simulink model "Speed_control"  (R2016b)
settings: Solver=VariableStepAuto  StartTime=0.0  StopTime=3  FixedStep=5e-6  RelTol=1e-3
libraries: powerlib x6, simulink x4, powerlib_meascontrol x3
settings Model: Creator=Awab Anwar  LastModifiedBy=Awab Anwar
settings DebuggingCC: MaxConsecutiveZCsMsg=none

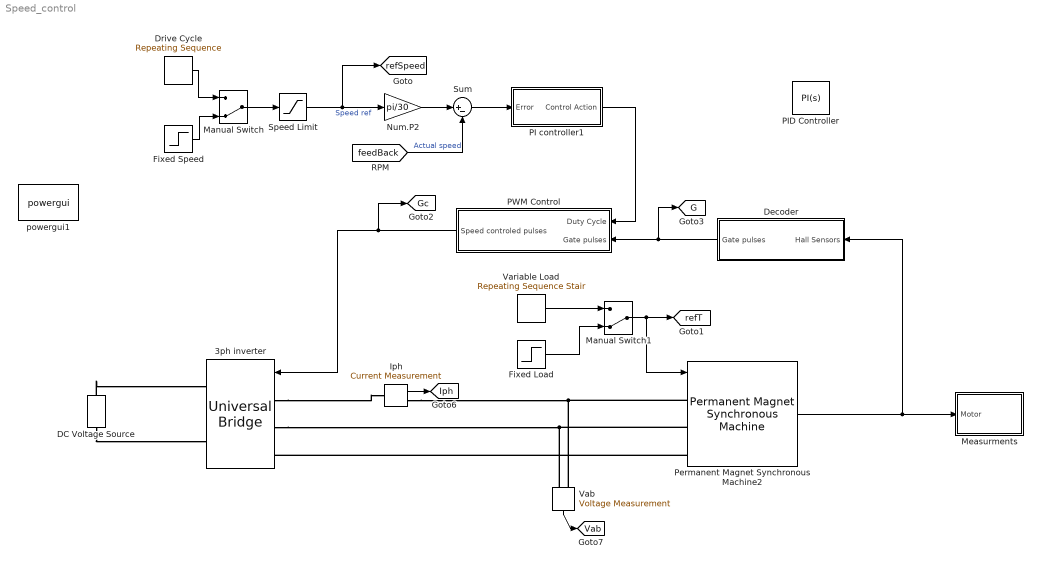
== system Speed_control ==
  3ph inverter : powerlib/Power Electronics/Universal Bridge  Arms=3  SnubberResistance=100  SnubberCapacitance=10e-6  Device=MOSFET / Diodes  Ron=0.000000001  Lon=0  ForwardVoltages="[  0  0  ]"  ForwardVoltage=0  GTOparameters=[ 10e-6 , 20e-6 ]  IGBTparameters=[ 1e-6 , 2e-6 ]  Measurements=Device voltages  Measurements_2=None  converterType=Rectifier
  DC Voltage Source : powerlib/Electrical Sources/DC Voltage Source  Amplitude=24  Measurements=None
  Decoder : Subsystem
  "Drive Cycle " : simulink/Sources/Repeating Sequence  rep_seq_t=[0 1 2 3 4 5 5.001 6 6.001 7]  rep_seq_y=[0 0 20 20 50 50 100 100 200 200]
  Fixed Speed : Step  Time=0  After=150  SampleTime=0
  Fixed Load : Step  Time=0  SampleTime=0
  Iph : powerlib/Measurements/Current Measurement  PhasorSimulation=off  OutputType=Complex  PSBequivalent=0
  Manual Switch : ManualSwitch  CurrentSetting=0
  Manual Switch1 : ManualSwitch  CurrentSetting=0
  Measurments : Subsystem
  Num.P2 : Gain  Gain=pi/30
  PI controller1 : Subsystem
  PID Controller : simulink/Continuous/PID Controller  Controller=PI  TimeDomain=Continuous-time  SampleTime=-1  IntegratorMethod=Forward Euler  FilterMethod=Forward Euler  Form=Parallel  UseFilter=on  ControllerParametersSource=internal  P=3  I=11.6  D=0  N=100  InitialConditionSource=internal  InitialConditionForIntegrator=0  InitialConditionForFilter=0  ExternalReset=none  LimitOutput=off  UpperSaturationLimit=inf  LowerSaturationLimit=-inf  LinearizeAsGain=on  AntiWindupMode=none  Kb=1  TrackingMode=off  Kt=1  PParamMin=[]  PParamMax=[]  IParamMin=[]  IParamMax=[]  DParamMin=[]  DParamMax=[]  NParamMin=[]  NParamMax=[]  KbParamMin=[]  KbParamMax=[]  KtParamMin=[]  KtParamMax=[]  POutMin=[]  POutMax=[]  IOutMin=[]  IOutMax=[]  DOutMin=[]  DOutMax=[]  NOutMin=[]  NOutMax=[]  KbOutMin=[]  KbOutMax=[]  KtOutMin=[]  KtOutMax=[]  IntegratorOutMin=[]  IntegratorOutMax=[]  FilterOutMin=[]  FilterOutMax=[]  SumOutMin=[]  SumOutMax=[]  SumI1OutMin=[]  SumI1OutMax=[]  SumI2OutMin=[]  SumI2OutMax=[]  SumI3OutMin=[]  SumI3OutMax=[]  SumDOutMin=[]  SumDOutMax=[]  SaturationOutMin=[]  SaturationOutMax=[]  IntegratorContinuousStateAttributes=''  IntegratorStateMustResolveToSignalObject=off  IntegratorRTWStateStorageClass=Auto  FilterContinuousStateAttributes=''  FilterStateMustResolveToSignalObject=off  FilterRTWStateStorageClass=Auto  DifferentiatorICPrevScaledInput=0  DifferentiatorOutMin=[]  DifferentiatorOutMax=[]
  PWM Control : Subsystem
  Permanent Magnet Synchronous Machine2 : powerlib/Machines/Permanent Magnet Synchronous Machine  NbPhases=3  FluxDistribution=Trapezoidal  RotorType=Round  MechanicalLoad=Torque Tm  PresetModel=No  ShowDetailedParameters=on  MeasurementBus=off  Resistance=0.25  Inductance=0.00025  dqInductances=[8.5e-3,8.5e-3]  La=0.0005  MachineConstant=Flux linkage established by magnets (V.s)  Flux=0.0222739  VoltageCst=93.3007  TorqueCst=0.89096  Flat=120  Mechanical=[0.2 0 20]  PolePairs=4  InitialConditions=[0,0, 0,0]  InitialConditions5ph=[0 0 0 0 0 0]  TsPowergui=0  TsBlock=-1  RefAngle=90 degrees behind phase A axis (modified Park)
  Speed Limit : Saturate  UpperLimit=150  LowerLimit=0
  Sum : Sum  Inputs=|+-
  Vab : powerlib/Measurements/Voltage Measurement  PhasorSimulation=off  OutputType=Complex  PSBequivalent=0
  "Variable Load " : simulink/Sources/Repeating Sequence Stair  OutValues=[1 3 5 8].'  tsamp=1  OutMin=[]  OutMax=[]  OutDataTypeStr=double  OutputDataTypeScalingMode=double  OutDataType=fixdt(0,8)  ConRadixGroup=Best Precision: Vector-wise  OutScaling=2^-12
  powergui1 : powerlib/powergui  Priority=1  SimulationMode=Discrete  SolverType=Tustin/Backward Euler (TBE)  SampleTime=5e-6  frequency=60  SPID=off  DisableSnubberDevices=off  DisableRonSwitches=off  DisableVfSwitches=off  SwTol=0  DisplayEquations=off  Interpol=off  ExternalGateDelay=off  methode=off  Ts=10  FunctionMessages=off  echomessages=off  HookPort=off  EnableUseOfTLC=off  x0status=blocks  frequencyindice=0  Pbase=100e6  ErrMax=1e-4  Iterations=50  UnitsV=kV  UnitsW=MW  buscounter=0  RestoreLinks=warning  ResistiveCurrentMeasurement=off  Frange=[0:2:500]  Ylog=off  Xlog=on  ShowGrid=off  save=off  variable=ZData  structure=0  ZoomFFT=off  StartTime=0.0  cycles=1  DisplayStyle=1  fundamental=60  FreqAxis=off  MaxFrequency=1000  frequencyindicesteady=1  RmsSteady=1  display=off
  tag scope: G=global, Gc=global, Iph=global, Vab=global, refSpeed=global, refT=global
  wires:
  Decoder/1(Gate pulses) -> [G], PWM Control/2(Gate pulses)
  PWM Control/1(Speed controled pulses) -> 3ph inverter/1, [Gc]
  [feedBack] -> Sum/2  "Actual speed"
  Sum/1 -> PI controller1/1(Error)
  Manual Switch/1 -> Speed Limit/1
  Speed Limit/1 -> [refSpeed], Num.P2/1  "Speed ref"
  Fixed Speed/1 -> Manual Switch/2
  Num.P2/1 -> Sum/1
  "Drive Cycle "/1 -> Manual Switch/1
  Permanent Magnet Synchronous Machine2/1 -> Decoder/1(Hall Sensors), Measurments/1(Motor)
  "Variable Load "/1 -> Manual Switch1/1
  Fixed Load/1 -> Manual Switch1/2
  Manual Switch1/1 -> Permanent Magnet Synchronous Machine2/1, [refT]
  Iph/1 -> [Iph]
  Vab/1 -> [Vab]
  PI controller1/1(Control Action) -> PWM Control/1(Duty Cycle)
  connections:
  Vab/LConn2 -- Permanent Magnet Synchronous Machine2/LConn2 -- 3ph inverter/LConn2
  Vab/LConn1 -- Permanent Magnet Synchronous Machine2/LConn1 -- Iph/RConn1
  Permanent Magnet Synchronous Machine2/LConn3 -- 3ph inverter/LConn3
  3ph inverter/LConn1 -- Iph/LConn1
  DC Voltage Source/RConn1 -- 3ph inverter/RConn1
  DC Voltage Source/LConn1 -- 3ph inverter/RConn2

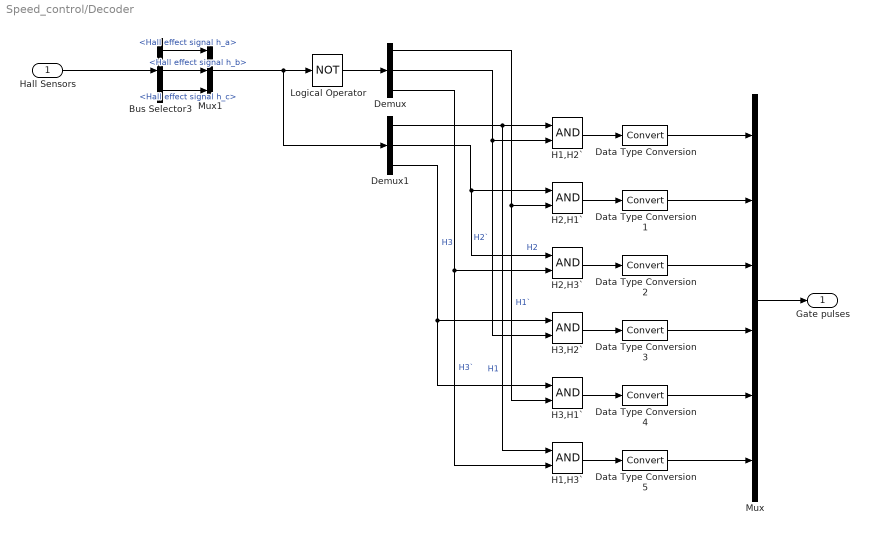
== system Speed_control/Decoder ==
  Hall Sensors : Inport
  Bus Selector3 : BusSelector  OutputSignals=Hall effect signal h_a,Hall effect signal h_b,Hall effect signal h_c
  Data Type Conversion{,1..5} (6 alike) : DataTypeConversion
  Demux : Demux  Outputs=3
  Demux1 : Demux  Outputs=3
  H1,H2` : Logic  AllPortsSameDT=off  OutDataTypeStr=boolean
  H1,H3` : Logic  AllPortsSameDT=off  OutDataTypeStr=boolean
  H2,H1` : Logic  AllPortsSameDT=off  OutDataTypeStr=boolean
  H2,H3` : Logic  AllPortsSameDT=off  OutDataTypeStr=boolean
  H3,H1` : Logic  AllPortsSameDT=off  OutDataTypeStr=boolean
  H3,H2` : Logic  AllPortsSameDT=off  OutDataTypeStr=boolean
  Logical Operator : Logic  Operator=NOT  AllPortsSameDT=off  OutDataTypeStr=boolean
  Mux : Mux  Inputs=6
  Mux1 : Mux  Inputs=3
  Gate pulses : Outport
  wires:
  Mux1/1 -> Demux1/1, Logical Operator/1
  Logical Operator/1 -> Demux/1
  Demux1/1 -> H1,H3`/1, H1,H2`/1  "H1"
  Demux1/2 -> H2,H3`/1, H2,H1`/1  "H2"
  Demux1/3 -> H3,H2`/1, H3,H1`/1  "H3"
  Demux/1 -> H3,H1`/2, H2,H1`/2  "H1`"
  Demux/2 -> H3,H2`/2, H1,H2`/2  "H2`"
  Demux/3 -> H2,H3`/2, H1,H3`/2  "H3`"
  H1,H2`/1 -> Data Type Conversion/1
  H2,H1`/1 -> Data Type Conversion1/1
  H2,H3`/1 -> Data Type Conversion2/1
  H3,H2`/1 -> Data Type Conversion3/1
  H3,H1`/1 -> Data Type Conversion4/1
  H1,H3`/1 -> Data Type Conversion5/1
  Mux/1 -> Gate pulses/1
  Data Type Conversion/1 -> Mux/1
  Data Type Conversion1/1 -> Mux/2
  Data Type Conversion2/1 -> Mux/3
  Data Type Conversion3/1 -> Mux/4
  Data Type Conversion4/1 -> Mux/5
  Data Type Conversion5/1 -> Mux/6
  Bus Selector3/3 -> Mux1/3  "<Hall effect signal h_c>"
  Bus Selector3/2 -> Mux1/2  "<Hall effect signal h_b>"
  Bus Selector3/1 -> Mux1/1  "<Hall effect signal h_a>"
  Hall Sensors/1 -> Bus Selector3/1

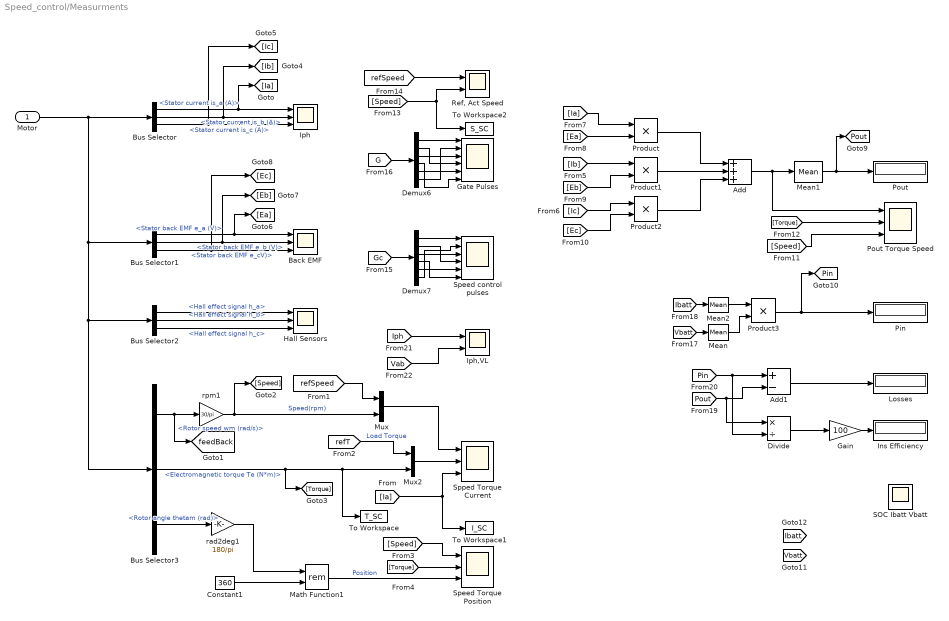
== system Speed_control/Measurments ==
  Motor : Inport
  Add : Sum  Inputs=+++
  Add1 : Sum  Inputs=+-
  Back EMF : Scope  NumInputPorts=3
  Bus Selector : BusSelector  OutputSignals=Stator current is_a (A),Stator current is_b (A),Stator current is_c (A)
  Bus Selector1 : BusSelector  OutputSignals=Stator back EMF e_a (V),Stator back EMF e_b (V),Stator back EMF e_cV)
  Bus Selector2 : BusSelector  OutputSignals=Hall effect signal h_a,Hall effect signal h_b,Hall effect signal h_c
  Bus Selector3 : BusSelector  OutputSignals=Rotor speed wm (rad/s),Electromagnetic torque Te (N*m),Rotor angle thetam (rad)
  Constant1 : Constant  Value=360
  Demux6 : Demux  Outputs=6
  Demux7 : Demux  Outputs=6
  Divide : Product  Inputs=*/
  Gain : Gain  Gain=100
  Gate Pulses : Scope  NumInputPorts=6
  "Hall Sensors " : Scope  NumInputPorts=3
  Ins Efficiency : Display
  Iph : Scope  NumInputPorts=3
  Iph,VL : Scope  NumInputPorts=2
  Losses : Display
  Math Function1 : Math  Operator=rem  SaturateOnIntegerOverflow=on
  Mean : powerlib_meascontrol/Measurements/Mean  Freq=60  Vinit=0  Ts=0
  Mean1 : powerlib_meascontrol/Measurements/Mean  Freq=60  Vinit=0  Ts=0
  Mean2 : powerlib_meascontrol/Measurements/Mean  Freq=60  Vinit=0  Ts=0
  Mux : Mux  Inputs=2
  Mux2 : Mux  Inputs=2
  Pin : Display
  Pout : Display
  Pout Torque Speed : Scope  NumInputPorts=3
  Product{,1..3} (4 alike) : Product
  "Ref, Act Speed" : Scope  NumInputPorts=2
  SOC Ibatt Vbatt : Scope  NumInputPorts=3
  Speed Torque Position : Scope  NumInputPorts=3
  Speed control pulses : Scope  NumInputPorts=6
  Spped Torque Current : Scope  NumInputPorts=3
  To Workspace : ToWorkspace  VariableName=T_SC  SaveFormat=Timeseries  SampleTime=-1
  To Workspace1 : ToWorkspace  VariableName=I_SC  SaveFormat=Timeseries  SampleTime=-1
  To Workspace2 : ToWorkspace  VariableName=S_SC  SaveFormat=Timeseries  SampleTime=-1
  rad2deg1 : Gain  Gain=180/pi
  rpm1 : Gain  Gain=30/pi
  tag scope: Ibatt=global, Pin=global, Pout=global, Vbatt=global, feedBack=global
  wires:
  Motor/1 -> Bus Selector3/1, Bus Selector2/1, Bus Selector1/1, Bus Selector/1
  Demux6/1 -> Gate Pulses/1
  Demux6/6 -> Gate Pulses/2
  Demux6/3 -> Gate Pulses/3
  Demux6/5 -> Gate Pulses/5
  Demux6/2 -> Gate Pulses/4
  Demux6/4 -> Gate Pulses/6
  Constant1/1 -> Math Function1/2
  rad2deg1/1 -> Math Function1/1
  Mux/1 -> Spped Torque Current/1
  Mux2/1 -> Spped Torque Current/2
  rpm1/1 -> [Speed], Mux/2  "Speed(rpm)"
  [Gc] -> Demux7/1
  Demux7/1 -> Speed control pulses/1
  Demux7/6 -> Speed control pulses/2
  Demux7/3 -> Speed control pulses/3
  Demux7/5 -> Speed control pulses/5
  Demux7/2 -> Speed control pulses/4
  Demux7/4 -> Speed control pulses/6
  Bus Selector/1 -> [Ia], Iph/1  "<Stator current is_a (A)>"
  Bus Selector/2 -> [Ib], Iph/2  "<Stator current is_b (A)>"
  Bus Selector/3 -> [Ic], Iph/3  "<Stator current is_c (A)>"
  Bus Selector3/1 -> [feedBack], rpm1/1  "<Rotor speed wm (rad/s)>"
  Bus Selector3/3 -> rad2deg1/1  "<Rotor angle thetam (rad)>"
  Bus Selector3/2 -> [Torque], To Workspace/1, Mux2/2  "<Electromagnetic torque Te (N*m)>"
  Bus Selector2/1 -> "Hall Sensors "/1  "<Hall effect signal h_a>"
  Bus Selector2/2 -> "Hall Sensors "/2  "<Hall effect signal h_b>"
  Bus Selector2/3 -> "Hall Sensors "/3  "<Hall effect signal h_c>"
  Bus Selector1/1 -> [Ea], Back EMF/1  "<Stator back EMF e_a (V)>"
  Bus Selector1/2 -> [Eb], Back EMF/2  "<Stator back EMF e_b (V)>"
  Bus Selector1/3 -> [Ec], Back EMF/3  "<Stator back EMF e_cV)>"
  [Ia] -> To Workspace1/1, Spped Torque Current/3
  [refSpeed] -> Mux/1
  [refT] -> Mux2/1  "Load Torque"
  Math Function1/1 -> Speed Torque Position/3  "Position"
  [Speed] -> Speed Torque Position/1
  [Torque] -> Speed Torque Position/2
  [Ia] -> Product/1
  [Ea] -> Product/2
  [Ib] -> Product1/1
  [Eb] -> Product1/2
  [Ic] -> Product2/1
  [Ec] -> Product2/2
  Product1/1 -> Add/2
  Product/1 -> Add/1
  Product2/1 -> Add/3
  Add/1 -> Mean1/1, Pout Torque Speed/1
  [Torque] -> Pout Torque Speed/2
  [Speed] -> Pout Torque Speed/3
  [refSpeed] -> "Ref, Act Speed"/1
  [Speed] -> To Workspace2/1, "Ref, Act Speed"/2
  [G] -> Demux6/1
  Product3/1 -> [Pin], Pin/1
  [Pin] -> Divide/2, Add1/1
  [Pout] -> Divide/1, Add1/2
  Add1/1 -> Losses/1
  Divide/1 -> Gain/1
  [Iph] -> Iph,VL/1
  [Vab] -> Iph,VL/2
  [Ibatt] -> Mean2/1
  Mean2/1 -> Product3/1
  [Vbatt] -> Mean/1
  Mean/1 -> Product3/2
  Gain/1 -> Ins Efficiency/1
  Mean1/1 -> [Pout], Pout/1

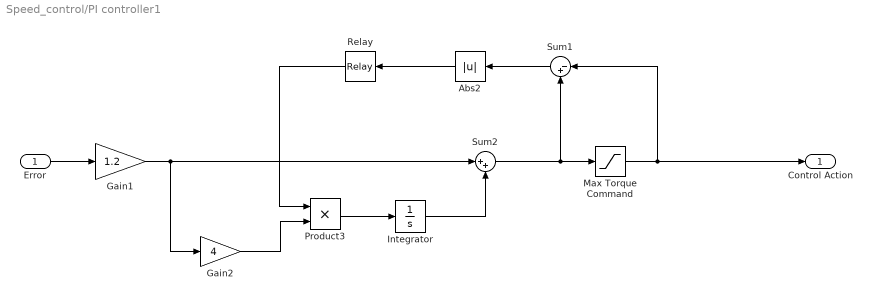
== system Speed_control/PI controller1 ==
  Error : Inport
  Abs2 : Abs  SaturateOnIntegerOverflow=on
  Gain1 : Gain  Gain=1.2
  Gain2 : Gain  Gain=4
  Integrator : Integrator
  Max Torque Command : Saturate  UpperLimit=1  LowerLimit=0
  Product3 : Product
  Relay : Relay  OffSwitchValue=0  OnOutputValue=0  OffOutputValue=1
  Sum1 : Sum  Inputs=|-+
  Sum2 : Sum  Inputs=|++
  Control Action : Outport
  wires:
  Sum1/1 -> Abs2/1
  Integrator/1 -> Sum2/2
  Error/1 -> Gain1/1
  Product3/1 -> Integrator/1
  Gain1/1 -> Gain2/1, Sum2/1
  Gain2/1 -> Product3/2
  Abs2/1 -> Relay/1
  Sum2/1 -> Max Torque Command/1, Sum1/2
  Max Torque Command/1 -> Control Action/1, Sum1/1
  Relay/1 -> Product3/1

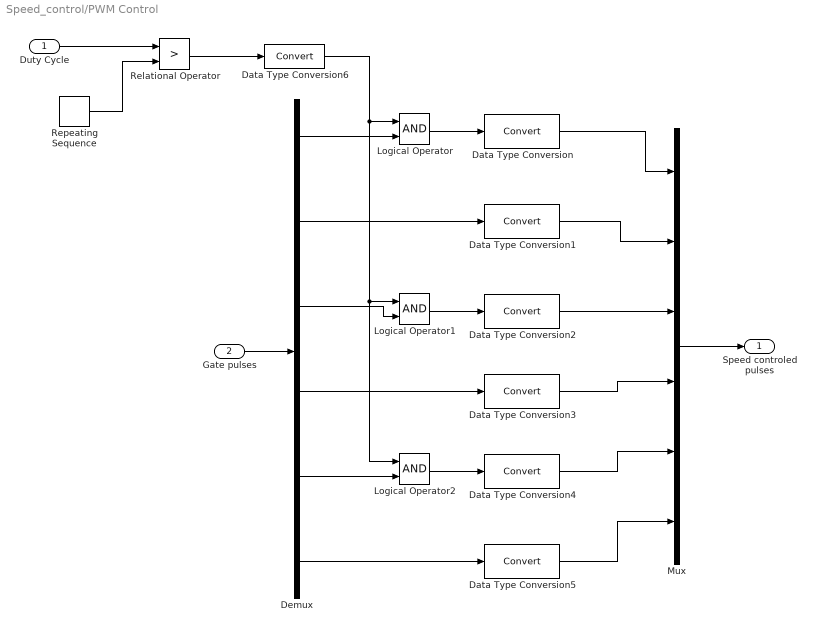
== system Speed_control/PWM Control ==
  Duty Cycle : Inport
  Gate pulses : Inport  Port=2
  Data Type Conversion{,1..6} (7 alike) : DataTypeConversion
  Demux : Demux  Outputs=6
  Logical Operator : Logic  AllPortsSameDT=off  OutDataTypeStr=boolean
  Logical Operator1 : Logic  AllPortsSameDT=off  OutDataTypeStr=boolean
  Logical Operator2 : Logic  AllPortsSameDT=off  OutDataTypeStr=boolean
  Mux : Mux  Inputs=6
  Relational Operator : RelationalOperator  Operator=>  OutDataTypeStr=boolean  RndMeth=Simplest
  Repeating Sequence : simulink/Sources/Repeating Sequence  rep_seq_t=[0 2e-4]  rep_seq_y=[0 1]
  Speed controled pulses : Outport
  wires:
  Data Type Conversion6/1 -> Logical Operator1/1, Logical Operator2/1, Logical Operator/1
  Repeating Sequence/1 -> Relational Operator/2
  Duty Cycle/1 -> Relational Operator/1
  Relational Operator/1 -> Data Type Conversion6/1
  Data Type Conversion5/1 -> Mux/6
  Data Type Conversion4/1 -> Mux/5
  Data Type Conversion3/1 -> Mux/4
  Data Type Conversion2/1 -> Mux/3
  Data Type Conversion1/1 -> Mux/2
  Data Type Conversion/1 -> Mux/1
  Mux/1 -> Speed controled pulses/1
  Demux/6 -> Data Type Conversion5/1
  Logical Operator2/1 -> Data Type Conversion4/1
  Demux/4 -> Data Type Conversion3/1
  Logical Operator1/1 -> Data Type Conversion2/1
  Demux/2 -> Data Type Conversion1/1
  Logical Operator/1 -> Data Type Conversion/1
  Demux/5 -> Logical Operator2/2
  Demux/3 -> Logical Operator1/2
  Demux/1 -> Logical Operator/2
  Gate pulses/1 -> Demux/1
